simulink model "on_line1"  (R2018a)
settings: Solver=VariableStepAuto  StartTime=0.0  StopTime=20  RelTol=1e-3
libraries: ctrlSharedLib x1
settings Model: Creator=Dominik  LastModifiedBy=Dominik

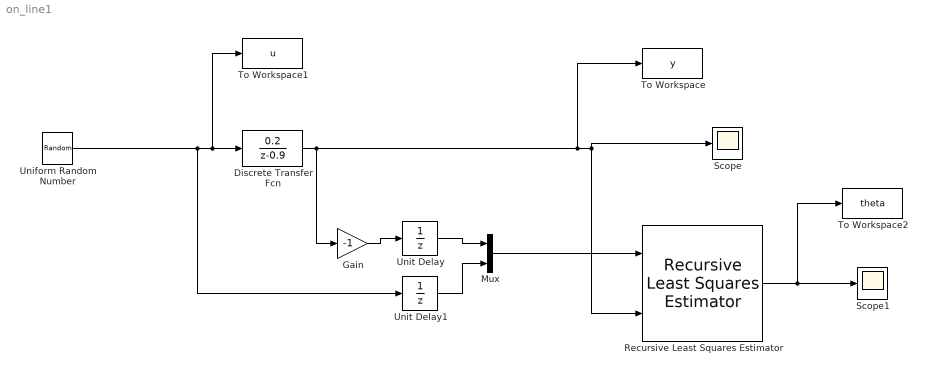
== system on_line1 ==
  Discrete Transfer Fcn : DiscreteTransferFcn  Numerator=[0.2]  Denominator=[1 -0.9]
  Gain : Gain  Gain=-1
  Mux : Mux  Inputs=2
  Recursive Least Squares Estimator : ctrlSharedLib/Recursive Least Squares Estimator  InitialEstimateSource=Internal  InitialParameterData=[1 1]  P0=10  EstimationMethod=Forgetting Factor  AdaptationParameter=1  HasTimeVaryingAdaptationParameter=off  NormalizationBias=eps  OutputError=off  OutputP=off  AddEnablePort=off  Ts=-1
      settings: SourceProductName=Control System Toolbox  SourceProductBaseCode=CT
  Scope : Scope
  Scope1 : Scope
  To Workspace : ToWorkspace  VariableName=y  SampleTime=-1
  To Workspace1 : ToWorkspace  VariableName=u  SampleTime=-1
  To Workspace2 : ToWorkspace  VariableName=theta  SampleTime=-1
  Uniform Random Number : UniformRandomNumber  SampleTime=0.1
  Unit Delay : UnitDelay  SampleTime=-1
  Unit Delay1 : UnitDelay  SampleTime=-1
  wires:
  Discrete Transfer Fcn/1 -> Gain/1, Scope/1, Recursive Least Squares Estimator/2, To Workspace/1
  Gain/1 -> Unit Delay/1
  Unit Delay/1 -> Mux/1
  Unit Delay1/1 -> Mux/2
  Uniform Random Number/1 -> To Workspace1/1, Discrete Transfer Fcn/1, Unit Delay1/1
  Mux/1 -> Recursive Least Squares Estimator/1
  Recursive Least Squares Estimator/1 -> To Workspace2/1, Scope1/1
